simulink model "TV_2017"  (R2016a)
settings: Solver=FixedStepAuto  StartTime=0.0  StopTime=inf  FixedStep=0.001  RelTol=1e-3
PreLoadFcn:
  | TV_2017_parameters
values from neighbouring files (symbols this model uses):
  battery_voltage = single(530)    [HIL_parameters.m]    (also in HIL_parameters_2018.m; TV_2017_parameters.m; TV_2017_parameters_VD.m)
  car_params = Simulink_Car_params    [HIL_parameters.m]    (also in HIL_parameters_2018.m; TV_2017_parameters.m; TV_2017_parameters_VD.m)
  i_Diff = 16    [HIL_parameters.m]    (also in HIL_parameters_2018.m; TV_2017_parameters.m)
  Kp = 1    [HIL_parameters.m]    (also in HIL_parameters_2018.m; TV_2017_parameters.m; TV_2017_parameters_VD.m)
  motor_data = struct    [HIL_parameters.m]    (also in HIL_parameters_2018.m; TV_2017_parameters.m)
  powerLimitControl = Simulink_el    [HIL_parameters.m]    (also in HIL_parameters_2018.m; TV_2017_parameters.m; TV_2017_parameters_VD.m)
  settings = Simulink_Settings    [HIL_parameters.m]    (also in HIL_parameters_2018.m; TV_2017_parameters.m; TV_2017_parameters_VD.m)
  SpdC_BCC = 0    [HIL_parameters.m]    (also in HIL_parameters_2018.m; TV_2017_parameters.m; TV_2017_parameters_VD.m)
  Speed_Neg_sat = -21    [HIL_parameters.m]    (also in HIL_parameters_2018.m; TV_2017_parameters.m; TV_2017_parameters_VD.m)
  Speed_Pos_sat = 21    [HIL_parameters.m]    (also in HIL_parameters_2018.m; TV_2017_parameters.m; TV_2017_parameters_VD.m)
  SteeringAngleFL = [-23.80 -22.65 -21.50 -20.34 -19.18 -18.03 -16.86 -15.70 -14.53 -13.35 -12.18 -10.99 -9.80 -8.61 -7.40 -6.19 -4.97 -3.75 -2.51 -1.26 0 1.27 2.56 3.85 5.17 6.50 7.84 9.21 10.59 12.00 13.42 14.88 16.36 17.87 19.41 20.99 22.61 24.26 25.97 27.73 29.54]    [CarSetupAnalysis2018.m]    (also in HIL_parameters_2018.m; TV_2017_parameters.m; TV_2017_parameters_VD.m = [-24.129 -22.950 -21.772 -20.593 -19.413 -18.232 -17.050 -15)
  SteeringAngleFR = [-29.54 -27.73 -25.97 -24.26 -22.61 -20.99 -19.41 -17.87 -16.36 -14.88 -13.42 -12.00 -10.59 -9.21 -7.84 -6.50 -5.17 -3.85 -2.56 -1.27 0 1.26 2.51 3.75 4.97 6.19 7.40 8.61 9.80 10.99 12.18 13.35 14.53 15.70 16.86 18.03 19.18 20.34 21.50 22.65 23.80]    [CarSetupAnalysis2018.m]    (also in HIL_parameters_2018.m; TV_2017_parameters.m; TV_2017_parameters_VD.m = [-29.3050 -27.5340 -25.8140 -24.1410 -22.5110 -20.9180 -19.3)
  SteeringWhAngle = [-105 -99.75 -94.5 -89.25 -84 -78.75 -73.5 -68.25 -63 -57.75 -52.5 -47.25 -42 -36.75 -31.5 -26.25 -21.0 -15.75 -10.5 -5.25 0.0 5.25 10.50 15.75 21.00 26.25 31.50 36.75 42.00 47.25 52.50 57.75  63.00 68.25 73.50 78.75 84.00 89.25 94.50 99.75 105.00]    [TV_2017_parameters_VD.m]
  Tn_n = 0    [HIL_parameters.m]    (also in HIL_parameters_2018.m; TV_2017_parameters.m; TV_2017_parameters_VD.m)
  tractionControl = Simulink_tc    [HIL_parameters.m]    (also in HIL_parameters_2018.m; IterativeTractionControlTuning.m; TV_2017_parameters.m; TV_2017_parameters_VD.m)
  yawMomentGenerator = struct    [HIL_parameters.m]    (also in HIL_parameters_2018.m = Simulink_yawRate2; TV_2017_parameters.m = Simulink_yawRate2)
  yawRateControl = Simulink_yawRate    [HIL_parameters.m]    (also in HIL_parameters_2018.m; TV_2017_parameters.m; TV_2017_parameters_VD.m)
undefined symbols (not defined in the file or in its folder): DiscIntNeverNeededParam, magnitude, speedEstimation, TC_Decr_Gas, TC_Derivative, TC_Incr_Gas, TC_On, TC_Relay_Off, TC_Relay_On
libraries: CarMaker4SL x350, simulink_extras x63, simulink x37, dspfdesign x2
(part 10 of 14)

== matlab function TV_2017/CarMaker/Control_System /Subsystem/Torque allocation 2017/Torque Allocation Quadratic Programming ==
  data: Mz_ref input; Ti_lim output Bus: Ti_lim; T_req input; states input; maxMotorTorque input; settings parameter; car_params parameter; yawRateControl parameter; saturated_constraints output; powerLimitControl parameter
function [Ti_lim, saturated_constraints] = QP(Mz_ref, T_req, states, maxMotorTorque, settings, car_params, yawRateControl, powerLimitControl)


max_matrix_dimention = 17;
Ti_max = [0 0 0 0];
Mz_allocated = single(0);
saturated_constraints = [0 0 0 0];
% ------- STATES -------------
r = states.r;
negative_torque_limit = yawRateControl.negative_torque_limit;

%---------- PARAMETERS -------
TV_method = settings.TV_Method;
mmt = single(settings.max_motor_torque);
mu = settings.mu;
lf = car_params.l_f;
lr = car_params.l_r;
tf = car_params.t_f;
tr = car_params.t_r;
arm_f = sqrt(tf^2 + lf^2);
GR = car_params.GR;
r_eff = car_params.r_eff;
R = [r_eff, r_eff, r_eff, r_eff]; % todo -> account for load
delta = states.wheel_angle;
delta_FL = delta;   % fix for later  ->individual steer angles
delta_FR = delta;
T_abs = abs(T_req); 
Mz_ref_scaled = Mz_ref * single(yawRateControl.enable);
pow_lim         = powerLimitControl.positive_power_limit; %= single(75000); % Positive effect limit
neg_pow_lim     = powerLimitControl.negative_power_limit;
error = 0;

rads_FL = max(10,abs(states.RPM_FL))*2*pi/60  *sign(states.RPM_FL);
rads_FR = max(10,abs(states.RPM_FR))*2*pi/60  *sign(states.RPM_FL);
rads_RL = max(10,abs(states.RPM_RL))*2*pi/60  *sign(states.RPM_FL);
rads_RR = max(10,abs(states.RPM_RR))*2*pi/60  *sign(states.RPM_FL);

mmt_FL = min(mmt, max(0.1, maxMotorTorque.mmt_FL));  % fix ned limit later
mmt_FR = min(mmt, max(0.1, maxMotorTorque.mmt_FR)); 
mmt_RL = min(mmt, max(0.1, maxMotorTorque.mmt_RL)); 
mmt_RR = min(mmt, max(0.1, maxMotorTorque.mmt_RR)); 
minmt_FL = min([mmt_FL settings.max_motor_brake_torque]);
minmt_FR = min([mmt_FR settings.max_motor_brake_torque]);
minmt_RL = min([mmt_RL settings.max_motor_brake_torque]);
minmt_RR = min([mmt_RR settings.max_motor_brake_torque]);
%***************************************************

M_T_FL =     GR/R(1) *  -sin(  atan(tf/lf)  -  delta_FL)  *arm_f;
M_T_FR =     GR/R(2) *   sin(  atan(tf/lf)  +  delta_FR)  *arm_f;
M_T_RL =     GR/R(3) *  -tr;
M_T_RR =     GR/R(4) *   tr;

%***************************************************

G_1       = 2*[ M_T_FL^2         ,          M_T_FL *M_T_FR   ,       M_T_FL*M_T_RL   ,        M_T_FL*M_T_RR    ;
               M_T_FR * M_T_FL    ,           M_T_FR^2        ,       M_T_FR*M_T_RL   ,        M_T_FR*M_T_RR    ;
               M_T_RL * M_T_FL    ,        M_T_RL*M_T_FR      ,         M_T_RL^2      ,        M_T_RL*M_T_RR    ;
               M_T_RR * M_T_FL    ,        M_T_RR*M_T_FR      ,      M_T_RR* M_T_RL   ,            M_T_RR^2  ];

G_2  =[        2/mmt_FL^2,    0,          0,          0;
                  0,      2/mmt_FR^2,     0,          0;
                  0,          0,      2/mmt_RL^2,     0;
                  0,          0,          0,      2/mmt_RR^2];
              
G_3 =[
    ];

G = G_1/100 + 100000*G_2;

c       = [M_T_FL  , M_T_FR  , M_T_RL  ,  M_T_RR    ]'*-2*Mz_ref_scaled;      

A_eq   =  single([ 1   1   1   1 ]);
b_eq   =  T_req ;

A      =     single([rads_FL ,   rads_FR ,   rads_RL ,    rads_RR   ;
                         1    ,       0    ,       0    ,        0      ;
                         0    ,       1    ,       0    ,        0      ;
                         0    ,       0    ,       1    ,        0      ;
                         0    ,       0    ,       0    ,        1      ;
                        -1    ,       0    ,       0    ,        0      ;
                         0    ,      -1    ,       0    ,        0      ;
                         0    ,       0    ,      -1    ,        0      ;
                         0    ,       0    ,       0    ,       -1      ]);

b    =  [pow_lim ,  mmt_FL  ,    mmt_FR  ,    mmt_RL  ,     mmt_RR    , mmt_FL  ,  mmt_FR  ,  mmt_RL  ,   mmt_RR ]'; 
% ------------------- POWLIM not done !! is done for now? compensate for efficiency later?`-------------------
%Determine feasible startingpoint  / scale problem
%function [b_eq, x_o]  = determine_feasible_startingpoint(A,b,b_eq,pow_lim,T)

if b_eq > 0
    beta = b_eq /(-b(2) -b(3) -b(4) -b(5));
elseif b_eq < 0 
    beta = b_eq /(-b(6) -b(7) -b(8) -b(9)); 
else
    beta = single(0);
end


if (beta < 1)&&(beta > 0.001) % a feasible startingpoint exists (considering b(2:end))
    x_0 = beta * [-b(2) -b(3) -b(4)  -b(5)]';
    pow = -A(1,:)*x_0;
    if pow>pow_lim
        b_eq = T_req * (pow_lim/pow);
        x_0 = x_0*(pow_lim/pow);
    end
    x = active_set(G,c,A,b,A_eq,b_eq,x_0);
   
elseif (beta > -1)&&(beta < -0.001) % a feasible startingpoint exists (considering b(2:end))
    x_0 = beta * [-b(6) -b(7) -b(8)  -b(9)]';
    pow = -A(1,:)*x_0;
    if pow>pow_lim
        b_eq = T_req * (pow_lim/pow);
        x_0 = x_0*(pow_lim/pow);
    end
    x = active_set(G,c,A,b,A_eq,b_eq,x_0);
   
   
elseif (beta >= 1) % a feasible startingpoint does not exist (considering b(2:end))
    x_0 = [ -b(2)   -b(3) -b(4)  -b(5)]'; 
    pow = -A(1,:)*x_0;
    if pow>pow_lim
        b_eq = T_req * (pow_lim/pow);
        x_0 = x_0*(pow_lim/pow);
    end
    x = x_0;
else
    x = zeros(4,1,'single'); %default case, should not happen
end




% add constraints active based on lambda
Mz_allocated = [M_T_FL  , M_T_FR  , M_T_RL  ,  M_T_RR  ]* x;
Ti_lim_struct    = struct;
Ti_lim_struct.FL = x(1); Ti_lim_struct.FR = x(2); Ti_lim_struct.RL = x(3); Ti_lim_struct.RR = x(4);
Ti_lim = Ti_lim_struct;
active_const = [0 0 0 0];
end

%Active set method for convex QP  ( pg 472 optreg ) 
function x = active_set(G,c,A,b,A_eq,b_eq,x_0)

%0) Formulate KKT matrix

%1) set w_0 to be a subset of the actiive constraints at x_o


W_i = zeros(1,size(A,1),'single'); % W_i lists indexes of A in W
x_k = x_0;
x = single(x_0);


debug_main_iteration = 1;
notdone = 1;
iteration_count = 0;

while notdone
    if iteration_count > 100;
        disp('iteration-count overflow!')
        notdone = 0;
        x = x_k;
    end
    
   
    [p_k, all_lambda_positive] = calc_p_and_eval_lambda(G,  c,  A,  b, A_eq,  b_eq, W_i,  x_k );
    
    
    %debug-----------------------------------------------------------
    
    [alpha,violating_indexes] = compute_alpha(A,b,x_k,p_k,W_i);
    de_bug2 = A*(x_k + alpha*p_k) - b;
    ansr = min(de_bug2);
    if ansr < -0.01
        fail = true;
    end
    
    [p_k, all_lambda_positive] = calc_p_and_eval_lambda(G,  c,  A,  b, A_eq,  b_eq, W_i,  x_k ); 
    %debug________________________________________________
    
    if sum(abs(p_k)) <= 0.01
        if all_lambda_positive; 
            x = x_k;
            notdone = 0;
           
        else
            W_i = exclude_most_negative_lambda_index(G,  c,  A,  b,  A_eq,  b_eq,  x_k , W_i);
            iteration_count = iteration_count + 1;
        end
    elseif sum(abs(p_k)) ~= 0
        [alpha,violating_indexes] = compute_alpha(A,b,x_k,p_k,W_i);
        x_k = x_k + alpha*p_k ;
        if alpha < 1 %indicates blocking constraints
%           disp('blocking constraints')
            disp(alpha)
            %add one of blocking constraints to W_k
            new_index = find(violating_indexes,1); %returns index of first non-0 value
            W_i(new_index) = 1;
            iteration_count = iteration_count + 1;
        else
             
            iteration_count = iteration_count + 1;
        end
    else
        
        x = x_k;
        iteration_count = 105;
    end
end

% make it based on lambda
end

function [p_val, all_lambda_positive] =  calc_p_and_eval_lambda(G,  c,  A,  b, A_eq,  b_eq, W_i, x_k )
[W,b_w] = construct_working_set(A,  b, A_eq , b_eq ,  W_i);    
[p, lagrangians] = solve_KKT(G,  c,  W,  b_w,  x_k );
p_val = p;
%all_lambda_positive = sum(sign(lagrangians)) == (sum(W_i)+1);% indicates all values are positivr ( sign(0) returns false, will this cause error on loosely active constraints?  edit:  yes it did ....

if length(lagrangians)==size(b_eq,1)
    all_lambda_positive = true;
else
    all_lambda_positive = min(lagrangians((length(b_eq)+1):end)) >= 0; % indicates all values are positive       
end
end

function W_i = exclude_most_negative_lambda_index(G,  c,  A,  b,  A_eq, b_eq,  x_k , W_i)
[W,b_w] = construct_working_set(A,  b, A_eq , b_eq , W_i);   
[~, lagrangians] = solve_KKT(G,  c,  W,  b_w,  x_k );
% identify most negative lagrangian / 1 negative is guarranteed to exist
            low_value = single(0);
            low_index = int8(1);
            for j = (length(b_eq)+1):length(lagrangians)
                if lagrangians(j) <= low_value
                    low_value = lagrangians(j);
                    low_index = int8(j-1);
                else
                    %skip
                end
            end
            k = find(W_i,low_index);
            if k(low_index) > length(W_i)
                r=9;
            end
            W_i(k(low_index)) = 0;
            %W_i(low_index) = 0; % exclude j from IandW
            % construct new working set
            %[W,b_w] = construct_working_set(A_eq, b_eq, A, W_i, b);
            % got out of range error, tried to access second nonzero
            % element in W_i when there only where one nonzero elemnt (pow lim )
end

function [p, lambda_s] = solve_KKT(G,  c,  A,  b,  x_k )  % A is the working set W 
    sol = zeros(4+size(A,1),1,'single');
    %   add error handling here? 
    %   G, A and K needs full rank for K to be invertable
    
    h =  A*x_k   -   b           ;
    g =  c       +   G*x_k       ;
    K = [G             A'        ;
         A        zeros(size(A,1),'single')];
    
    sol      =   K\[g ; h];
    p        =   -sol(1:size(G,1));
    lambda_s =    sol((size(G,1)+1):size(G,1)+size(A,1));
end
 
function [alpha,violating_indexes] = compute_alpha(A, b , x_k , p_k ,  W_i) %% this is wrong, observed alpha -368.3450
    
    violating_indexes = zeros(1,size(A,1));
    values = ones(1,size(A,1));
    debug_values = ones(1,size(A,1));
    for i =  1:size(A,1) 
        if ~W_i(i)  &&  (A(i,:)*p_k < 0)
            val = (b(i) - A(i,:)*x_k)/(A(i,:)*p_k);
            debug_values(i) = val;
            if 0<=val && val<=1
                values(i) = val;
                violating_indexes(i) = 1;
            end
        else
            %skip
        end
    end
    alpha = min([1,values]);
end

function [W,b_w] = construct_working_set(A , b, A_eq , b_eq  , W_i )
W_ineq = zeros( dim_bound(sum(W_i)) , dim_bound(size(A_eq,2)) , 'single' ); 
b_ineq = zeros( dim_bound(sum(W_i)) , 1 , 'single' );
working_set_iterator = 1;
for u=1:size(A,1)
        if W_i(u)==1
            
            W_ineq(working_set_iterator,:) = A(u,:);
            b_ineq(working_set_iterator,1) = b(u);
            working_set_iterator = working_set_iterator + 1;
        end
end
W = [A_eq ; W_ineq]; 
b_w = [b_eq;b_ineq];
end

function y = dim_bound(n)
assert (n <= 17);
y = n;
end

== matlab function TV_2017/CarMaker/Control_System /Subsystem/Torque allocation 2017/max combined tire torque based on (Fz, SA,mu)  ==
  data: states input; maxMotorTorque output Bus: maxMotorTorque; settings parameter; car_params parameter; tractionControl parameter
function maxMotorTorque = maxTireForce(states,settings,car_params,tractionControl)
%#codegen
% draft scale function     (-x^4-x^2)/3 + -x^6/3  + 1
% calculate max tire force based on F_z and slip angle


% Need to be over a certain velocity for this to work....

v_x = states.V_x;
mu = settings.mu;
GR = car_params.GR;
r = car_params.r_eff;
max_slip = tractionControl.slip_ang_limit;
mmt = settings.max_motor_torque;

F_z_FL = states.Fz_FL;
F_z_FR = states.Fz_FR;
F_z_RL = states.Fz_RL;
F_z_RR = states.Fz_RR;

SA_norm_FL = states.SA_FL/max_slip;
SA_norm_FR = states.SA_FR/max_slip;
SA_norm_RL = states.SA_RL/max_slip;
SA_norm_RR = states.SA_RR/max_slip;

mu_scale_factor_FL = (-SA_norm_FL^4 -SA_norm_FL^2)/3 + -SA_norm_FL^6/3  + 1;
mu_scale_factor_FR = (-SA_norm_FR^4 -SA_norm_FR^2)/3 + -SA_norm_FR^6/3  + 1;
mu_scale_factor_RL = (-SA_norm_RL^4 -SA_norm_RL^2)/3 + -SA_norm_RL^6/3  + 1;
mu_scale_factor_RR = (-SA_norm_RR^4 -SA_norm_RR^2)/3 + -SA_norm_RR^6/3  + 1;

if v_x > 2;
    maxMotorTorque.mmt_FL = F_z_FL * mu_scale_factor_FL *mu * r/ GR ;
    maxMotorTorque.mmt_FR = F_z_FR * mu_scale_factor_FR *mu * r/ GR ;
    maxMotorTorque.mmt_RL = F_z_RL * mu_scale_factor_RL *mu * r/ GR ;
    maxMotorTorque.mmt_RR = F_z_RR * mu_scale_factor_RR *mu * r/ GR ;
else
    maxMotorTorque.mmt_FL = mmt;
    maxMotorTorque.mmt_FR = mmt;
    maxMotorTorque.mmt_RL = mmt;
    maxMotorTorque.mmt_RR = mmt;
end

end

== matlab function TV_2017/CarMaker/Control_System /Subsystem/Torque allocation 2017/max long tire torque based on (FZ , mu) ==
  data: states input; maxMotorTorque output Bus: maxMotorTorque; settings parameter; car_params parameter
function maxMotorTorque = maxTireForce(states,settings, car_params)
%#codegen

% calculate max tire force based on F_z and slip angle
mu = settings.mu;
GR = car_params.GR;
r = car_params.r_eff;

F_z_FL = states.Fz_FL;
F_z_FR = states.Fz_FR;
F_z_RL = states.Fz_RL;
F_z_RR = states.Fz_RR;


maxMotorTorque.mmt_FL = F_z_FL * r * mu / GR ;
maxMotorTorque.mmt_FR = F_z_FR * r * mu / GR ;
maxMotorTorque.mmt_RL = F_z_RL * r * mu / GR ;
maxMotorTorque.mmt_RR = F_z_RR * r * mu / GR ;

== matlab function TV_2017/CarMaker/Control_System /Subsystem/Torque allocation 2017/max torque  ==
  data: mu_lim input; SA_lim input; maxMotorTorque output Bus: maxMotorTorque; active_constraints output; inv_temp_lim input; mot_temp_lim input; settings parameter
function [maxMotorTorque, active_constraints] = maxTireForce(mu_lim,SA_lim,inv_temp_lim,mot_temp_lim, settings)
%#codegen
active_constraints = zeros(1,(6*4),'int8');

default_max_torque = settings.max_motor_torque;
default_min_torque = settings.max_motor_brake_torque;
%calc_pow_lim.mmt_FL,
FL_max = max(0,min([inv_temp_lim.mmt_FL,mot_temp_lim.mmt_FL,mu_lim.mmt_FL,SA_lim.mmt_FL,default_max_torque]));
FR_max = max(0,min([inv_temp_lim.mmt_FR,mot_temp_lim.mmt_FR,mu_lim.mmt_FR,SA_lim.mmt_FR,default_max_torque]));
RL_max = max(0,min([inv_temp_lim.mmt_RL,mot_temp_lim.mmt_RL,mu_lim.mmt_RL,SA_lim.mmt_RL,default_max_torque]));
RR_max = max(0,min([inv_temp_lim.mmt_RR,mot_temp_lim.mmt_RR,mu_lim.mmt_RR,SA_lim.mmt_RR,default_max_torque]));

maxMotorTorque.mmt_FL = FL_max;
maxMotorTorque.mmt_FR = FR_max;
maxMotorTorque.mmt_RL = RL_max;
maxMotorTorque.mmt_RR = RR_max;

i = 1;
% active_constraints(i) = isequal(calc_pow_lim.mmt_FL,FL_max); i = i+1;
% active_constraints(i) = isequal(calc_pow_lim.mmt_FR,FR_max); i = i+1;
% active_constraints(i) = isequal(calc_pow_lim.mmt_RL,RL_max); i = i+1;
% active_constraints(i) = isequal(calc_pow_lim.mmt_RR,RR_max); i = i+1;
default_lim_FL = isequal(default_max_torque,FL_max);   %returns 1 if default max torque is the active limit
default_lim_FR = isequal(default_max_torque,FR_max);
default_lim_RL = isequal(default_max_torque,RL_max);
default_lim_RR = isequal(default_max_torque,RR_max);

active_constraints(i) = default_lim_FL;  i = i+1;
active_constraints(i) = default_lim_FR;  i = i+1;
active_constraints(i) = default_lim_RL;  i = i+1;
active_constraints(i) = default_lim_RR;  i = i+1;
% Available power
active_constraints(i) = 0;%isequal(calc_pow_lim.mmt_FL,FL_max) *(1- default_lim_FL) ; i = i+1;
active_constraints(i) = 0;%isequal(calc_pow_lim.mmt_FR,FR_max) *(1- default_lim_FR) ; i = i+1;
active_constraints(i) = 0;%isequal(calc_pow_lim.mmt_RL,RL_max) *(1- default_lim_RL) ; i = i+1;
active_constraints(i) = 0;%isequal(calc_pow_lim.mmt_RR,RR_max) *(1- default_lim_RR) ; i = i+1;
% Inverter temperature
active_constraints(i) = isequal(inv_temp_lim.mmt_FL,FL_max) *(1- default_lim_FL) ;  i = i+1;
active_constraints(i) = isequal(inv_temp_lim.mmt_FR,FR_max) *(1- default_lim_FR) ;  i = i+1;
active_constraints(i) = isequal(inv_temp_lim.mmt_RL,RL_max) *(1- default_lim_RL) ;  i = i+1;
active_constraints(i) = isequal(inv_temp_lim.mmt_RR,RR_max) *(1- default_lim_RR) ;  i = i+1;
%Motor temperature
active_constraints(i) = isequal(mot_temp_lim.mmt_FL,FL_max) *(1- default_lim_FL) ;  i = i+1;
active_constraints(i) = isequal(mot_temp_lim.mmt_FR,FR_max) *(1- default_lim_FR) ;  i = i+1;
active_constraints(i) = isequal(mot_temp_lim.mmt_RL,RL_max) *(1- default_lim_RL) ;  i = i+1;
active_constraints(i) = isequal(mot_temp_lim.mmt_RR,RR_max) *(1- default_lim_RR) ;  i = i+1;
% Friction square
active_constraints(i) = isequal(mu_lim.mmt_FL,FL_max) *(1- default_lim_FL) ;  i = i+1;
active_constraints(i) = isequal(mu_lim.mmt_FR,FR_max) *(1- default_lim_FR) ;  i = i+1;
active_constraints(i) = isequal(mu_lim.mmt_RL,RL_max) *(1- default_lim_RL) ;  i = i+1;
active_constraints(i) = isequal(mu_lim.mmt_RR,RR_max) *(1- default_lim_RR) ;  i = i+1;
% friction ellipse
active_constraints(i) = isequal(SA_lim.mmt_FL,FL_max) *(1- default_lim_FL) ;  i = i+1;
active_constraints(i) = isequal(SA_lim.mmt_FR,FR_max) *(1- default_lim_FR) ;  i = i+1;
active_constraints(i) = isequal(SA_lim.mmt_RL,RL_max) *(1- default_lim_RL) ;  i = i+1;
active_constraints(i) = isequal(SA_lim.mmt_RR,RR_max) *(1- default_lim_RR) ;  i = i+1;


%active_constraints(i) = i;  i = i+1;
 

%active_constraints

== matlab function TV_2017/CarMaker/Control_System /Subsystem/Torque allocation 2017/maxMotorTorque and kers based on available power ==
  data: states input; maxMotorTorque output Bus: maxMotorTorque; settings parameter; kers_allowed output
function [maxMotorTorque,kers_allowed] = MaxMotorTorque_Power(states,settings)
%#codegen

% DC Voltage                             / states
% Max allowable current draw in total    /settings
% Load distribution                      /states






if states.V_x<=settings.KERS_speed_limit_hyst_low
    kers_allowed = single(0);
elseif states.V_x>=settings.KERS_speed_limit_hyst_high
    kers_allowed = single(1);
else
    kers_allowed = single(0);
end

Fzi = [max(1,states.Fz_FL) max(1,states.Fz_FR) max(1,states.Fz_RL) max(1,states.Fz_RR)]';

switch settings.TV_Method
    case 1 % No negative torque
        alfa_r =  (Fzi(3) + Fzi(4)) / (Fzi(1) + Fzi(2) + Fzi(3) + Fzi(4));
    case 2 % with negative torque
        alfa_r =  (Fzi(3) + Fzi(4)) / (Fzi(1) + Fzi(2) + Fzi(3) + Fzi(4));
    case 3 % static 25 %
        alfa_r = single(0.5);
    case 4 % with negative torque, no Fz
        alfa_r = single(0.5);
    otherwise
        alfa_r = single(0.5);
end

RPM_to_angular = single(2*pi/60);
omega_FL = states.RPM_FL*RPM_to_angular;
omega_FR = states.RPM_FR*RPM_to_angular;
omega_RL = states.RPM_RL*RPM_to_angular;
omega_RR = states.RPM_RR*RPM_to_angular;

mmt = settings.max_motor_torque;
available_power = states.DC_voltage*settings.max_battery_discharge;

max_torque_front = min(mmt, (available_power*(1-alfa_r))/ (2 * max( max(1,omega_FL), max(1,omega_FR))) );
max_torque_rear = min(mmt, (available_power*alfa_r)     / (2 * max( max(1,omega_RL), max(1,omega_RR))) );
                      
maxMotorTorque.mmt_FL = max_torque_front;
maxMotorTorque.mmt_FR = max_torque_front;
maxMotorTorque.mmt_RL = max_torque_rear;
maxMotorTorque.mmt_RR = max_torque_rear;

== matlab function TV_2017/CarMaker/Control_System /Power Limit Torque Reduction Controller 2018/Old powerlimiting /extractPower1 ==
  data: states input; power output; powerLimitControl parameter
function power = extractPower(states,powerLimitControl)
%#codegen


if (powerLimitControl.enable == uint32(1))
    power = states.power;
else
    power = single(0);
end

end
